simulink subsystem "GyroIntegrator"  (R2021a)
settings: Solver=VariableStepAuto  StartTime=0.0  StopTime=10.0  RelTol=1e-3
undefined symbols (not defined in the file): q0
libraries: aerolibutil x1
settings Model: Creator=Laura  LastModifiedBy=Laura

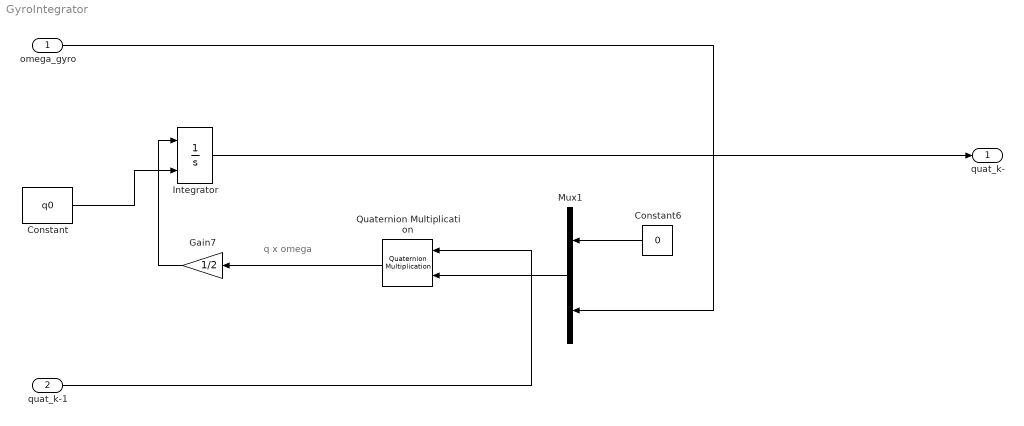
== system GyroIntegrator ==
  note: q x omega
  omega_gyro : Inport
  quat_k-1 : Inport  Port=2
  Constant : Constant  Value=q0
  Constant6 : Constant  Value=0
  Gain7 : Gain  Gain=1/2
  Integrator : Integrator  InitialConditionSource=external
  Mux1 : Mux  Inputs=2
  Quaternion Multiplication : aerolibutil/Quaternion Multiplication
  quat_k- : Outport
  wires:
  Gain7/1 -> Integrator/1
  Quaternion Multiplication/1 -> Gain7/1
  omega_gyro/1 -> Mux1/2
  Mux1/1 -> Quaternion Multiplication/2
  Constant6/1 -> Mux1/1
  Constant/1 -> Integrator/2
  quat_k-1/1 -> Quaternion Multiplication/1
  Integrator/1 -> quat_k-/1
